simulink model "Lab07A"  (R2021a)
settings: Solver=VariableStepAuto  StartTime=0.0  StopTime=50  RelTol=1e-3
libraries: simulink x1
settings Model: Creator=levivandek  LastModifiedBy=levivandek

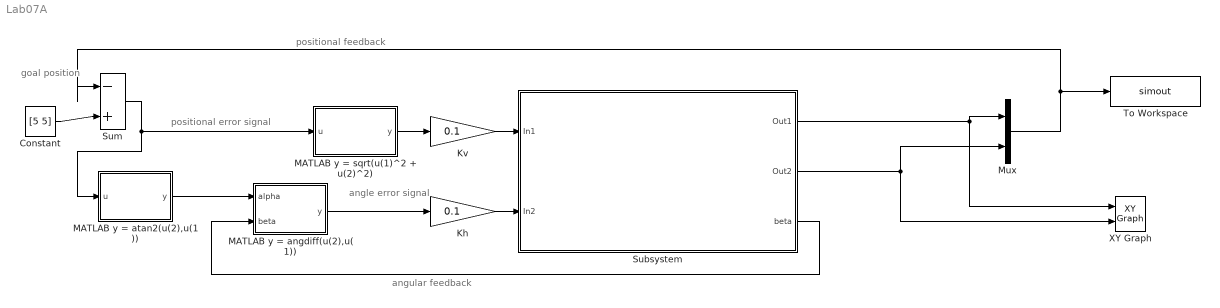
== system Lab07A ==
  note: positional error signal
  note: goal
      | position
  note: angle
      | error signal
  note: positional feedback
  note: angular feedback
  Constant : Constant  Value=[5 5]
  Kh : Gain  Gain=0.1
  Kv : Gain  Gain=0.1
  MATLAB y = angdiff(u(2),u(1)) : MATLAB Function  TreatAsAtomicUnit=on
  MATLAB y = atan2(u(2),u(1)) : MATLAB Function  TreatAsAtomicUnit=on
  MATLAB y = sqrt(u(1)^2 + u(2)^2) : MATLAB Function  TreatAsAtomicUnit=on
  Mux : Mux  Inputs=2
  Subsystem : Subsystem
  Sum : Sum  Inputs=|-+
  To Workspace : ToWorkspace  VariableName=simout  SaveFormat=Timeseries  SampleTime=-1
  XY Graph : simulink/Sinks/XY Graph  xmin=0  xmax=8  ymin=0  ymax=11  st=-1
  wires:
  Kv/1 -> Subsystem/1(In1)
  Kh/1 -> Subsystem/2(In2)
  Subsystem/2(Out2) -> Mux/2, XY Graph/2
  Subsystem/1(Out1) -> XY Graph/1, Mux/1
  Mux/1 -> Sum/1, To Workspace/1
  Subsystem/3(beta) -> MATLAB y = angdiff(u(2),u(1))/2(beta)
  MATLAB y = angdiff(u(2),u(1))/1(y) -> Kh/1
  MATLAB y = sqrt(u(1)^2 + u(2)^2)/1(y) -> Kv/1
  MATLAB y = atan2(u(2),u(1))/1(y) -> MATLAB y = angdiff(u(2),u(1))/1(alpha)
  Sum/1 -> MATLAB y = atan2(u(2),u(1))/1(u), MATLAB y = sqrt(u(1)^2 + u(2)^2)/1(u)
  Constant/1 -> Sum/2

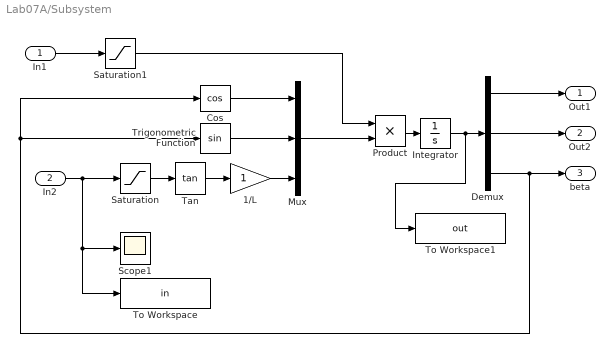
== system Lab07A/Subsystem ==
  In1 : Inport
  In2 : Inport  Port=2
  1/L : Gain
  Cos : Trigonometry  Operator=cos
  Demux : Demux  Outputs=3
  Integrator : Integrator  InitialCondition=[8 5 pi/2]
  Mux : Mux  Inputs=3
  Product : Product
  Saturation : Saturate  UpperLimit=1  LowerLimit=-1
  Saturation1 : Saturate  UpperLimit=1  LowerLimit=-1
  Scope1 : Scope
  Tan : Trigonometry  Operator=tan
  To Workspace : ToWorkspace  VariableName=in  SaveFormat=Timeseries  SampleTime=-1
  To Workspace1 : ToWorkspace  VariableName=out  SaveFormat=Timeseries  SampleTime=-1
  Trigonometric Function : Trigonometry
  Out1 : Outport
  Out2 : Outport  Port=2
  beta : Outport  Port=3
  wires:
  Cos/1 -> Mux/1
  Demux/1 -> Out1/1
  In2/1 -> Scope1/1, To Workspace/1, Saturation/1
  1/L/1 -> Mux/3
  Product/1 -> Integrator/1
  Integrator/1 -> To Workspace1/1, Demux/1
  Saturation1/1 -> Product/1
  In1/1 -> Saturation1/1
  Saturation/1 -> Tan/1
  Trigonometric Function/1 -> Mux/2
  Demux/3 -> Cos/1, Trigonometric Function/1, beta/1
  Demux/2 -> Out2/1
  Mux/1 -> Product/2
  Tan/1 -> 1/L/1

== matlab function Lab07A/MATLAB y = angdiff(u(2),u(1)) ==
  data: alpha input; y output; beta input
function y= fcn(alpha, beta)

    gama=alpha-beta;

    if abs(gama)>2*pi
        gama1=gama-fix(gama/2/pi)*2*pi; %removes the decimals
    else
        gama1=gama;
    end

    if abs(gama1)>pi
       if gama1>0
           y=gama1-2*pi;
       else
           y=gama1+2*pi;
       end
    else
        y=gama1;
    end

end

== matlab function Lab07A/MATLAB y = atan2(u(2),u(1)) ==
  data: u input; y output
function y = fcn(u)

y = atan2(u(2),u(1));

== matlab function Lab07A/MATLAB y = sqrt(u(1)^2 + u(2)^2) ==
  data: u input; y output
function y = fcn(u)

y = sqrt(u(1)^2 + u(2)^2);
